simulink model "pil_topmodel_stm32f7"  (R2018b)
settings: Solver=FixedStepDiscrete  StartTime=0.0  StopTime=1000  RelTol=1e-3  EnableMultiTasking=on
PostLoadFcn:
  | init_model()
undefined symbols (not defined in the file or in its folder): DiscIntNeverNeededParam
settings Model: Creator=mbussjaeger  LastModifiedBy=csax
settings DataIOCC: LimitDataPoints=on  SaveFormat=Array  SignalLoggingSaveFormat=ModelDataLogs
settings OptimizationCC: DefaultParameterBehavior=Inlined  EnhancedBackFolding=on  PassReuseOutputArgsAs=Individual arguments  ExpressionDepthLimit=2147483647  OptimizeBlockOrder=speed  DifferentSizesBufferReuse=on  OptimizationCustomize=off
settings DebuggingCC: UnderspecifiedInitializationDetection=Classic  MergeDetectMultiDrivingBlocksExec=none  SolverPrmCheckMsg=warning  ParameterTunabilityLossMsg=error  FcnCallInpInsideContextMsg=warning  AllowSymbolicDim=off  StateNameClashWarn=warning  SFUnexpectedBacktrackingDiag=warning  SFNoUnconditionalDefaultTransitionDiag=warning  SFExecutionAtInitializationDiag=none
settings HardwareCC: ProdBitPerPointer=32  ProdBitPerSizeT=32  ProdBitPerPtrDiffT=32  ProdLargestAtomicInteger=Long  ProdLargestAtomicFloat=Double  ProdWordSize=32  ProdHWDeviceType=ARM Compatible->ARM Cortex
settings ModelReferenceCC: UpdateModelReferenceTargets=IfOutOfDate  PropagateSignalLabelsOutOfModel=off
settings SFSimCC: SimUseLocalCustomCode=off  MATLABDynamicMemAlloc=off
settings RTWCC: SystemTargetFile=ert.tlc  TemplateMakefile=ert_default_tmf  RTWUseLocalCustomCode=off  Toolchain=TRACE32 XIL GCC arm-none-eabi Cortex-M | gmake makefile  IncludeHyperlinkInReport=on
settings CodeAppCC: ForceParamTrailComments=on  IgnoreCustomStorageClasses=off  OperatorAnnotations=on  SimulinkDataObjDesc=on  SFDataObjDesc=on  InsertBlockDesc=on
settings ERTTargetCC: GenerateSampleERTMain=on  InlinedParameterPlacement=NonHierarchical  ERTCustomFileTemplate=example_file_process.tlc
settings ConfigComp: CovMetricSettings=dw  CovHtmlReporting=on  CovSaveCumulativeToWorkspaceVar=on  CovSaveSingleToWorkspaceVar=on  CovExternalEMLEnable=off  CovSFcnEnable=off

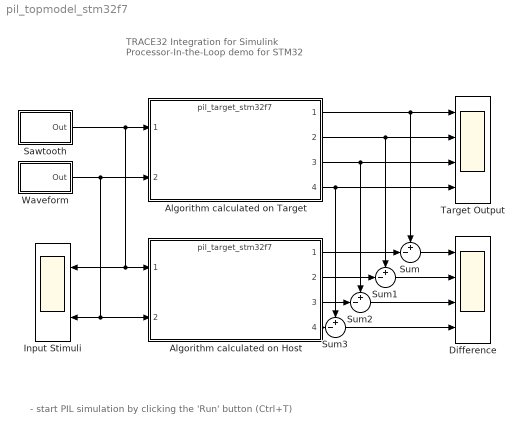
== system pil_topmodel_stm32f7 ==
  note: TRACE32 Integration for Simulink
      | Processor-In-the-Loop demo for STM32
  note: - start PIL simulation by clicking the 'Run' button (Ctrl+T)
  Algorithm calculated on Host : ModelReference  ModelNameDialog=pil_target_stm32f7.slx  SimulationMode=Normal  ModelReferenceVersion=1.56
  Algorithm calculated on Target : ModelReference  ModelNameDialog=pil_target_stm32f7.slx  SimulationMode=Processor-in-the-loop (PIL)  ModelReferenceVersion=1.56
  Difference : Scope  NumInputPorts=4
  Input Stimuli : Scope  NumInputPorts=2
  Sawtooth : Subsystem
  Sum{,1..3} (4 alike) : Sum  Inputs=+-|
  Target Output : Scope  NumInputPorts=4
  Waveform : Subsystem
  wires:
  Sawtooth/1(Out) -> Algorithm calculated on Target/1, Input Stimuli/1, Algorithm calculated on Host/1
  Waveform/1(Out) -> Algorithm calculated on Target/2, Input Stimuli/2, Algorithm calculated on Host/2
  Algorithm calculated on Target/4 -> Target Output/4, Sum3/1
  Algorithm calculated on Target/3 -> Target Output/3, Sum2/1
  Algorithm calculated on Target/2 -> Target Output/2, Sum1/1
  Algorithm calculated on Target/1 -> Target Output/1, Sum/1
  Sum/1 -> Difference/1
  Sum1/1 -> Difference/2
  Sum2/1 -> Difference/3
  Sum3/1 -> Difference/4
  Algorithm calculated on Host/1 -> Sum/2
  Algorithm calculated on Host/4 -> Sum3/2
  Algorithm calculated on Host/3 -> Sum2/2
  Algorithm calculated on Host/2 -> Sum1/2

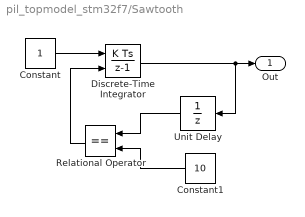
== system pil_topmodel_stm32f7/Sawtooth ==
  Constant : Constant  OutDataTypeStr=uint16
  Constant1 : Constant  Value=10  OutDataTypeStr=uint16
  Discrete-Time Integrator : DiscreteIntegrator  ExternalReset=rising  ICPrevOutput=DiscIntNeverNeededParam  ICPrevScaledInput=DiscIntNeverNeededParam
  Relational Operator : RelationalOperator  Operator===  OutDataTypeStr=boolean  RndMeth=Nearest
  Unit Delay : UnitDelay  SampleTime=-1
  Out : Outport
  wires:
  Constant/1 -> Discrete-Time Integrator/1
  Discrete-Time Integrator/1 -> Unit Delay/1, Out/1
  Relational Operator/1 -> Discrete-Time Integrator/2
  Unit Delay/1 -> Relational Operator/1
  Constant1/1 -> Relational Operator/2

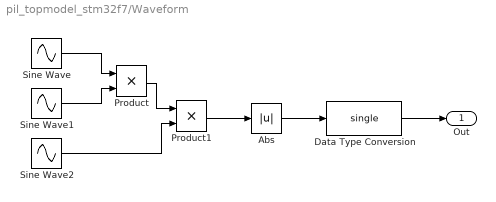
== system pil_topmodel_stm32f7/Waveform ==
  Abs : Abs
  Data Type Conversion : DataTypeConversion  OutDataTypeStr=single
  Product : Product  RndMeth=Zero
  Product1 : Product  RndMeth=Zero
  Sine Wave : Sin  SineType=Sample based  Amplitude=3.14159265359  Samples=1000  SampleTime=1
  Sine Wave1 : Sin  SineType=Sample based  Amplitude=31.4159265359  Samples=333  SampleTime=1
  Sine Wave2 : Sin  SineType=Sample based  Amplitude=0.314159265359  Samples=777  SampleTime=1
  Out : Outport
  wires:
  Sine Wave/1 -> Product/1
  Sine Wave1/1 -> Product/2
  Sine Wave2/1 -> Product1/2
  Product/1 -> Product1/1
  Product1/1 -> Abs/1
  Abs/1 -> Data Type Conversion/1
  Data Type Conversion/1 -> Out/1
